simulink model "Model"  (R2019b)
settings: Solver=VariableStepAuto  StartTime=0.0  StopTime=10  RelTol=1e-3
values from neighbouring files (symbols this model uses):
  A = [u_j ; v_j ; w_j ; p_j ; q_j ; r_j ; x_j ; y_j ; z_j ; phi_j ; theta_j ; psi_j]    [LimSim7.m]
  B = [u_j ; v_j ; w_j ; p_j ; q_j ; r_j ; x_j ; y_j ; z_j ; phi_j ; theta_j ; psi_j]    [LimSim7.m]
  C = [h_j ; ax_j ; ay_j ; az_j]    [LimSim7.m]
  D = [h_j ; ax_j ; ay_j ; az_j]    [LimSim7.m]
  K_R = lqr(A_R, B_R, Q_R, R_R)    [LimSim7.m]
  M = [1, 1,    1, -1 ... (first row only)    [LimSim7.m]
  R = diag([1])    [LimSim7.m]
  tau1 = 30/1000    (= 0.03)    [LimSim7.m]
  tau2 = 1/10    (= 0.1)    [LimSim7.m]
libraries: sharedutil x4, vrlib x2, aerolibutil x1, simulink x1
settings Model: Creator=ethan  LastModifiedBy=ethan

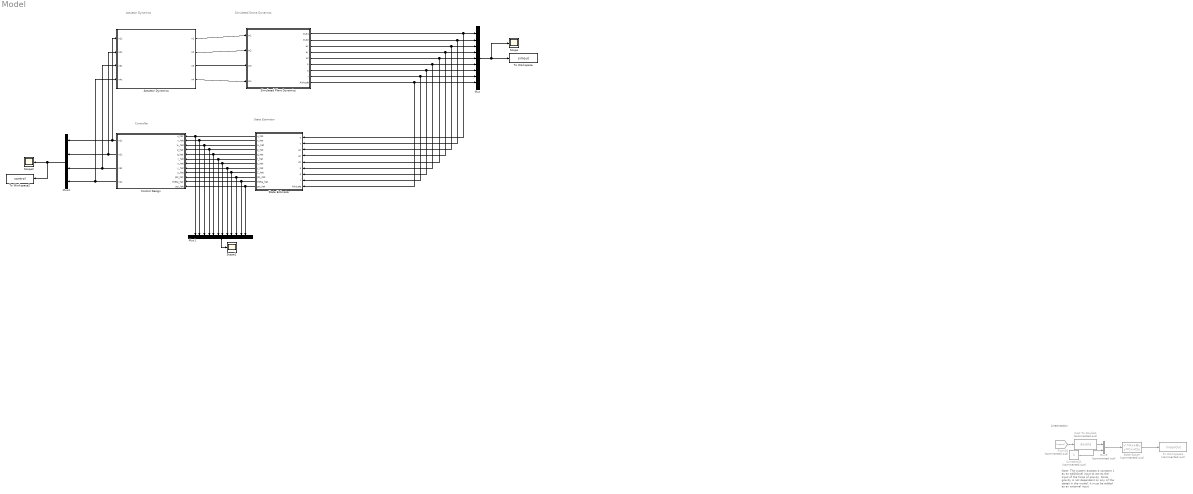
== system Model ==
  note: Actuator Dynamics
  note: Note: The system accepts a constant 1 as an additional input to act as the input of the force of gravity. Since gravity is not dependent on any of the states in the model, it must be added as an external input
  note: Linearization
  note: Simulated Drone Dynamics
  note: State Estimator
  note: Controller
  "Actuator Dynamics " : Subsystem
  Cast To Double1 : DataTypeConversion  Commented=on  OutDataTypeStr=double
  Constant21 : Constant  Commented=on
  Control Design : Subsystem
  From26 : From  Commented=on  GotoTag=motors
  Mux : Mux  Inputs=9
  Mux1 : Mux  Inputs=12
  Mux2 : Mux
  Mux9 : Mux  Commented=on  Inputs=2
  Scope : Scope
  Scope1 : Scope
  Scope2 : Scope
  Simulated Plant Dynamics : Subsystem
  State Estimator : Subsystem
  State-Space : StateSpace  Commented=on  A=A  B=B  C=C  D=D  InitialCondition=[0,0,0,0,0,0,0,0,0,0,0,0]
  To Workspace : ToWorkspace  VariableName=simout  SaveFormat=Structure With Time  SampleTime=-1
  To Workspace1 : ToWorkspace  Commented=on  VariableName=linearOut  SaveFormat=Timeseries  SampleTime=-1
  To Workspace2 : ToWorkspace  VariableName=control  SaveFormat=Timeseries  SampleTime=-1
  wires:
  State-Space/1 -> To Workspace1/1
  Constant21/1 -> Mux9/2
  Cast To Double1/1 -> Mux9/1
  From26/1 -> Cast To Double1/1
  Mux9/1 -> State-Space/1
  "Actuator Dynamics "/2(n2) -> Simulated Plant Dynamics/2(In2)
  "Actuator Dynamics "/1(n1) -> Simulated Plant Dynamics/1(In1)
  "Actuator Dynamics "/3(n3) -> Simulated Plant Dynamics/3(In3)
  "Actuator Dynamics "/4(n4) -> Simulated Plant Dynamics/4(In4)
  Simulated Plant Dynamics/1(Out1) -> Mux/1, State Estimator/1(u)
  Simulated Plant Dynamics/2(Out2) -> Mux/2, State Estimator/2(v)
  Simulated Plant Dynamics/3(ax) -> Mux/3, State Estimator/3(ax)
  Simulated Plant Dynamics/4(ay) -> Mux/4, State Estimator/4(ay)
  Simulated Plant Dynamics/5(az) -> State Estimator/5(az), Mux/5
  Simulated Plant Dynamics/6(p) -> State Estimator/6(p), Mux/6
  Simulated Plant Dynamics/7(q) -> Mux/7, State Estimator/7(q)
  Simulated Plant Dynamics/8(r) -> State Estimator/8(r), Mux/8
  Simulated Plant Dynamics/9(Altitude) -> State Estimator/9(Altitude), Mux/9
  State Estimator/1(u_hat) -> Mux1/1, Control Design/1(u_hat)
  State Estimator/2(v_hat) -> Mux1/2, Control Design/2(v_hat)
  State Estimator/3(w_hat) -> Control Design/3(w_hat), Mux1/3
  State Estimator/4(p_hat) -> Control Design/4(p_hat), Mux1/4
  State Estimator/5(q_hat) -> Control Design/5(q_hat), Mux1/5
  State Estimator/6(r_hat) -> Mux1/6, Control Design/6(r_hat)
  State Estimator/7(x_hat) -> Mux1/7, Control Design/7(x_hat)
  State Estimator/8(y_hat) -> Mux1/8, Control Design/8(y_hat)
  State Estimator/9(Z_hat) -> Mux1/9, Control Design/9(z_hat)
  State Estimator/10(phi_hat) -> Mux1/10, Control Design/10(phi_hat)
  State Estimator/11(theta_hat) -> Control Design/11(theta_hat), Mux1/11
  State Estimator/12(psi_hat) -> Control Design/12(psi_hat), Mux1/12
  Control Design/1(n1c) -> "Actuator Dynamics "/1(n1c), Mux2/1
  Control Design/2(n2c) -> "Actuator Dynamics "/2(n2c), Mux2/2
  Control Design/3(n3c) -> "Actuator Dynamics "/3(n3c), Mux2/3
  Control Design/4(n4c) -> Mux2/4, "Actuator Dynamics "/4(n4c)
  Mux/1 -> Scope/1, To Workspace/1
  Mux1/1 -> Scope1/1
  Mux2/1 -> To Workspace2/1, Scope2/1

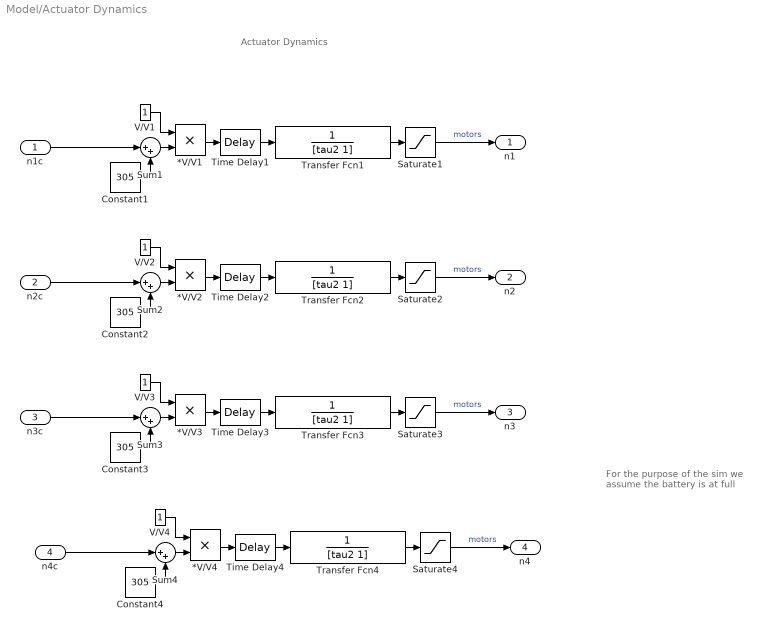
== system Model/Actuator Dynamics  ==
  note: For the purpose of the sim we assume the battery is at full
  note: Actuator Dynamics
  n1c : Inport
  n2c : Inport  Port=2
  n3c : Inport  Port=3
  n4c : Inport  Port=4
  *V/V{1..4} (4 alike) : Product
  Constant{1..4} (4 alike) : Constant  Value=305
  Saturate{1..4} (4 alike) : Saturate  UpperLimit=500  LowerLimit=10  OutDataTypeStr=single
  Sum{1..4} (4 alike) : Sum  Inputs=|++
  Time Delay{1..4} (4 alike) : TransportDelay  DelayTime=tau1
  Transfer Fcn{1..4} (4 alike) : TransferFcn  Denominator=[tau2 1]
  V/V{1..4} (4 alike) : Constant
  n1 : Outport
  n2 : Outport  Port=2
  n3 : Outport  Port=3
  n4 : Outport  Port=4
  wires:
  Transfer Fcn1/1 -> Saturate1/1
  n1c/1 -> Sum1/1
  Time Delay1/1 -> Transfer Fcn1/1
  Constant1/1 -> Sum1/2
  *V/V1/1 -> Time Delay1/1
  Sum1/1 -> *V/V1/2
  Saturate1/1 -> n1/1  "motors"
  V/V1/1 -> *V/V1/1
  Time Delay2/1 -> Transfer Fcn2/1
  Transfer Fcn2/1 -> Saturate2/1
  Constant2/1 -> Sum2/2
  Saturate2/1 -> n2/1  "motors"
  V/V2/1 -> *V/V2/1
  Sum2/1 -> *V/V2/2
  *V/V2/1 -> Time Delay2/1
  n2c/1 -> Sum2/1
  Time Delay3/1 -> Transfer Fcn3/1
  Transfer Fcn3/1 -> Saturate3/1
  Constant3/1 -> Sum3/2
  Saturate3/1 -> n3/1  "motors"
  V/V3/1 -> *V/V3/1
  Sum3/1 -> *V/V3/2
  *V/V3/1 -> Time Delay3/1
  n3c/1 -> Sum3/1
  Time Delay4/1 -> Transfer Fcn4/1
  Transfer Fcn4/1 -> Saturate4/1
  Constant4/1 -> Sum4/2
  Saturate4/1 -> n4/1  "motors"
  V/V4/1 -> *V/V4/1
  Sum4/1 -> *V/V4/2
  *V/V4/1 -> Time Delay4/1
  n4c/1 -> Sum4/1

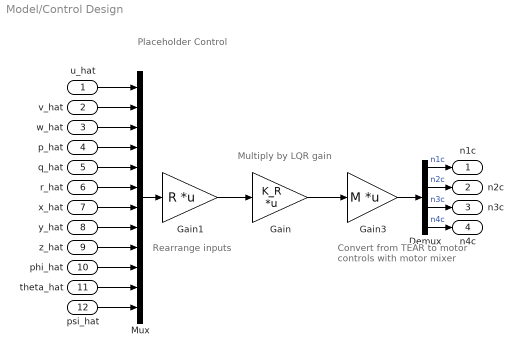
== system Model/Control Design ==
  note: Rearrange inputs
  note: Placeholder Control
  note: Multiply by LQR gain
  note: Convert from TEAR to motor controls with motor mixer
  u_hat : Inport
  v_hat : Inport  Port=2
  w_hat : Inport  Port=3
  p_hat : Inport  Port=4
  q_hat : Inport  Port=5
  r_hat : Inport  Port=6
  x_hat : Inport  Port=7
  y_hat : Inport  Port=8
  z_hat : Inport  Port=9
  phi_hat : Inport  Port=10
  theta_hat : Inport  Port=11
  psi_hat : Inport  Port=12
  Demux : Demux
  Gain : Gain  Gain=K_R  Multiplication=Matrix(K*u)
  Gain1 : Gain  Gain=R  Multiplication=Matrix(K*u)
  Gain3 : Gain  Gain=M  Multiplication=Matrix(K*u)
  Mux : Mux  Inputs=12
  n1c : Outport
  n2c : Outport  Port=2
  n3c : Outport  Port=3
  n4c : Outport  Port=4
  wires:
  Demux/1 -> n1c/1  "n1c"
  Demux/4 -> n4c/1  "n4c"
  theta_hat/1 -> Mux/11
  x_hat/1 -> Mux/7
  y_hat/1 -> Mux/8
  q_hat/1 -> Mux/5
  w_hat/1 -> Mux/3
  Demux/2 -> n2c/1  "n2c"
  p_hat/1 -> Mux/4
  Demux/3 -> n3c/1  "n3c"
  r_hat/1 -> Mux/6
  z_hat/1 -> Mux/9
  u_hat/1 -> Mux/1
  v_hat/1 -> Mux/2
  phi_hat/1 -> Mux/10
  psi_hat/1 -> Mux/12
  Mux/1 -> Gain1/1
  Gain1/1 -> Gain/1
  Gain/1 -> Gain3/1
  Gain3/1 -> Demux/1

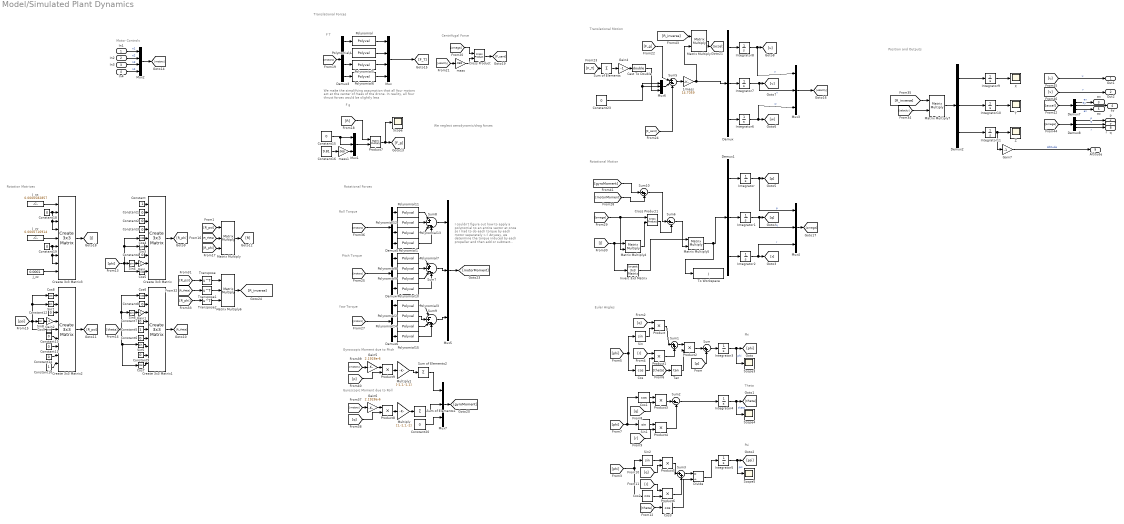
== system Model/Simulated Plant Dynamics ==
  note: I couldn't figure out how to apply a polynomial to an entire vector at once so I had to do each torque by each motor separately >:(
      |
      | Anyway, we determine the torque induced by each propeller and then add or subtract them accordingly to get the total torque about each axis
  note: We make the simplifying assumption that all four motors act at the center of mass of the drone. In reality, all four thrust forces would be slightly less
  note: Phi
  note: Motor Controls
  note: Translational Forces
  note: Euler Angles
  note: Rotation Matrices
  note: Theta
  note: Psi
  note: F g
  note: F T
  note: Translational Motion
  note: Rotational Motion
  note: Centrifugal Force
  note: Rotational Forces
  note: Pitch Torque
  note: Roll Torque
  note: Yaw Torque
  note: Gyroscopic Moment due to Pitch
  note: Gyroscopic Moment due to Roll
  note: Position and Outputs
  note: We neglect aerodynamic/drag forces
  In1 : Inport
  In2 : Inport  Port=2
  In3 : Inport  Port=3
  In4 : Inport  Port=4
  1/mass : Gain  Gain=14.7059
  Cast To Double : DataTypeConversion  OutDataTypeStr=double
  Constant : Constant
  Constant{1..4,6..9,11..15,18..20,23} (17 alike) : Constant  Value=0
  Constant10 : Constant
  Constant16 : Constant  Value=9.81
  Constant5 : Constant
  Cos{,1..9} (10 alike) : Trigonometry  Operator=cos
  Create 3x3 Matrix{,1..3} (4 alike) : sharedutil/Create 3x3 Matrix  aMode=aMode
  Cross Product : vrlib/Utilities/Cross Product
      settings: SourceProductName=Simulink
  Cross Product1 : vrlib/Utilities/Cross Product
      settings: SourceProductName=Simulink
  Demux{,1..2,7..8} (5 alike) : Demux  Outputs=3
  Demux{3..6} (4 alike) : Demux
  Divide : Product  Inputs=*/
  Gain{,1..2,4,7} (5 alike) : Gain  Gain=-1
  Gain5 : Gain  Gain=2.1928e-6
  Gain6 : Gain  Gain=2.1928e-6
  Integrator : Integrator  InitialCondition=rand/100
  Integrator{1..11} (11 alike) : Integrator
  Invert 3x3 Matrix : aerolibutil/Invert  3x3 Matrix
  J_xx : Constant  Value=0.0000582857
  J_yy : Constant  Value=0.0000716914
  J_zz : Constant  Value=0.0001
  Matrix Multiply : Product  Inputs=3  Multiplication=Matrix(*)
  Matrix Multiply{1,4..5,7} (4 alike) : Product  Multiplication=Matrix(*)
  Matrix Multiply6 : Product  Inputs=3  Multiplication=Matrix(*)
  Multiply : Gain  Gain=[1,-1,1,-1]
  Multiply1 : Gain  Gain=[-1,1,-1,1]
  Mux : Mux
  Mux{1,3..7} (6 alike) : Mux  Inputs=3
  Mux2 : Mux
  Polynomial{,4..6} (4 alike) : Polyval  Coefs=[ 1.066e-9 1.468e-6 0 0]
  Polynomial{1,7..13} (8 alike) : Polyval  Coefs=[ 5.07683e-11 6.99135e-8 0 0 ]
  Polynomial{2..3,14..15} (4 alike) : Polyval  Coefs="[  8.890e-9 0 0 ]"
  Product{,1..6,8..9} (9 alike) : Product
  Product7 : Product  Multiplication=Matrix(*)
  Scope{,3..5} (4 alike) : Scope
  Sin{,1..8} (9 alike) : Trigonometry
  Sum{,1,3,10} (4 alike) : Sum  Inputs=|++
  Sum of Elements : Sum  Inputs=+
  Sum of Elements1 : Sum  Inputs=+
  Sum of Elements2 : Sum  Inputs=+
  Sum2 : Sum  Inputs=|+-
  Sum5 : Sum  Inputs=|++-
  Sum6 : Sum  Inputs=|+-
  Sum7 : Sum  Inputs=|++--
  Sum8 : Sum  Inputs=|+--+
  Sum9 : Sum  Inputs=|-+-+
  Tan : Trigonometry  Operator=tan
  To Workspace : ToWorkspace  VariableName=j  SaveFormat=Structure  SampleTime=-1
  Transpose : Math  Operator=transpose  SignedPower=off  SaturateOnIntegerOverflow=on
  Transpose1 : Math  Operator=transpose  SignedPower=off  SaturateOnIntegerOverflow=on
  Transpose2 : Math  Operator=transpose  SignedPower=off  SaturateOnIntegerOverflow=on
  X : Scope
  Y : Scope
  Z : Scope
  mass : Gain  Gain=.068
  mass1 : Gain  Gain=.068
  Out1 : Outport
  Out2 : Outport  Port=2
  ax : Outport  Port=3
  ay : Outport  Port=4
  az : Outport  Port=5
  p : Outport  Port=6
  q : Outport  Port=7
  r : Outport  Port=8
  Altitude : Outport  Port=9
  wires:
  [omega] -> Demux8/1
  Product1/1 -> Sum1/2
  Polynomial7/1 -> Sum7/1
  Demux8/2 -> q/1  "q"
  Demux7/1 -> ax/1  "ax"
  In1/1 -> Mux2/1  "n1"
  Sin7/1 -> Create 3x3 Matrix2/2
  Integrator5/1 -> Scope5/1, [psi]  "psi"
  Sum10/1 -> Sum6/1
  [phi] -> Cos5/1, Cos4/1, Sin3/1, Sin4/1
  Gain4/1 -> Cast To Double/1
  Sum8/1 -> Mux5/1
  Create 3x3 Matrix/1 -> [R_phi]
  Integrator8/1 -> Mux3/1, [u]  "u"
  Constant5/1 -> Create 3x3 Matrix1/5
  Polynomial/1 -> Mux/1
  [phi] -> Cos/1, Sin/1
  Sum7/1 -> Mux5/2
  Constant20/1 -> Mux7/3
  Sin5/1 -> Create 3x3 Matrix1/7
  Demux5/3 -> Polynomial13/1
  Demux3/2 -> Polynomial4/1
  Product6/1 -> Sum3/2
  In4/1 -> Mux2/4  "n4"
  [phi] -> Sin1/1, Cos1/1
  Matrix Multiply1/1 -> [accel]
  Demux7/2 -> ay/1  "ay"
  Cos2/1 -> Product6/2
  Constant4/1 -> Create 3x3 Matrix/7
  Mux1/1 -> Product7/2
  Sin8/1 -> Gain2/1
  [v] -> Out2/1  "v"
  [F_cent] -> Sum5/3
  [theta] -> Cos6/1, Sin6/1, Cos7/1, Sin5/1
  Create 3x3 Matrix2/1 -> [R_psi]
  Product4/1 -> Sum2/2
  Polynomial13/1 -> Sum8/3
  Polynomial15/1 -> Sum9/4
  Constant3/1 -> Create 3x3 Matrix/4
  [p] -> Sum/2
  Product8/1 -> Multiply/1
  Constant13/1 -> Create 3x3 Matrix2/6
  Constant15/1 -> Mux1/2, Mux1/1
  Integrator6/1 -> Mux3/3, [w]  "w"
  Constant/1 -> Create 3x3 Matrix/1
  [r] -> Product4/2
  Constant9/1 -> Create 3x3 Matrix1/8
  1/mass/1 -> Matrix Multiply1/2, Demux/1
  [psi] -> Cos9/1, Cos8/1, Sin7/1, Sin8/1
  Constant2/1 -> Create 3x3 Matrix/3
  Product3/1 -> Sum2/1
  Integrator4/1 -> Scope4/1, [theta]  "theta"
  Sum5/1 -> 1/mass/1
  Cos6/1 -> Create 3x3 Matrix1/1
  Cos1/1 -> Product3/1
  [q] -> Product3/2
  [phi] -> Sin2/1, Cos2/1
  [q] -> Product8/2
  Integrator/1 -> Mux4/1, [p]  "p"
  Sin3/1 -> Create 3x3 Matrix/6
  Sum1/1 -> Product2/1
  [r] -> Product6/1
  Demux7/3 -> az/1  "az"
  Constant16/1 -> mass1/1
  [motors] -> Gain5/1
  Demux4/4 -> Polynomial10/1
  [q] -> Product5/2
  [motors] -> Demux6/1
  Sum of Elements/1 -> Gain4/1
  [theta] -> Cos3/1
  Integrator1/1 -> Mux4/2, [q]  "q"
  Sin6/1 -> Gain1/1
  Sum3/1 -> Divide/1
  Cos8/1 -> Create 3x3 Matrix2/1
  Constant1/1 -> Create 3x3 Matrix/2
  Product2/1 -> Sum/1
  Gain/1 -> Create 3x3 Matrix/8
  Integrator2/1 -> Mux4/3, [r]  "r"
  Transpose2/1 -> Matrix Multiply6/3
  J_yy/1 -> Create 3x3 Matrix3/5
  Product5/1 -> Sum3/1
  Integrator3/1 -> Scope3/1, [phi]  "phi"
  Gain1/1 -> Create 3x3 Matrix1/3
  Constant8/1 -> Create 3x3 Matrix1/2
  Gain6/1 -> Product8/1
  [R] -> Product7/1
  [R_phi] -> Matrix Multiply/3
  Constant14/1 -> Create 3x3 Matrix2/8
  Polynomial3/1 -> Sum9/1
  Matrix Multiply5/1 -> To Workspace/1, Demux1/1
  [R_psi] -> Matrix Multiply/1
  Cross Product/1 -> [F_cent]
  Matrix Multiply/1 -> [R]
  Constant10/1 -> Create 3x3 Matrix2/9
  Sin4/1 -> Gain/1
  Demux/3 -> Integrator6/1
  [theta] -> Tan/1
  Cos9/1 -> Create 3x3 Matrix2/5
  Sum2/1 -> Integrator4/1
  Mux4/1 -> [omega]
  Matrix Multiply7/1 -> Demux2/1
  Product/1 -> Sum1/1
  Gain2/1 -> Create 3x3 Matrix2/4
  Mux3/1 -> [velocity]
  Constant19/1 -> Create 3x3 Matrix3/8, Create 3x3 Matrix3/7, Create 3x3 Matrix3/6
  Polynomial6/1 -> Mux/4
  Polynomial1/1 -> Sum8/4
  [omega] -> Cross Product/1
  J_xx/1 -> Create 3x3 Matrix3/1
  J_zz/1 -> Create 3x3 Matrix3/9
  Sin2/1 -> Product5/1
  Product7/1 -> Scope/1, [F_g]
  Create 3x3 Matrix3/1 -> [J]
  [q] -> Product/1
  [R_theta] -> Transpose1/1
  Cos7/1 -> Create 3x3 Matrix1/9
  Multiply/1 -> Sum of Elements1/1
  Matrix Multiply6/1 -> [R_inverse]
  [F_g] -> Sum5/1
  Polynomial9/1 -> Sum7/3
  [R_phi] -> Transpose2/1
  Cos4/1 -> Create 3x3 Matrix/5
  Demux1/2 -> Integrator1/1
  [motorMoment] -> Sum10/2
  [r] -> Product1/1
  Invert 3x3 Matrix/1 -> Matrix Multiply5/1
  Constant12/1 -> Create 3x3 Matrix2/3
  Demux2/3 -> Integrator11/1
  Constant6/1 -> Create 3x3 Matrix1/6
  Demux3/3 -> Polynomial5/1
  [R_inverse] -> Matrix Multiply7/1
  Polynomial4/1 -> Mux/2
  [accel] -> Demux7/1
  Constant7/1 -> Create 3x3 Matrix1/4
  [velocity] -> mass/1
  Demux/1 -> Integrator8/1
  Mux/1 -> [F_T]
  Demux8/1 -> p/1  "p"
  [motors] -> Demux3/1
  Matrix Multiply4/1 -> Cross Product1/2
  Demux4/3 -> Polynomial9/1
  Create 3x3 Matrix1/1 -> [R_theta]
  Demux3/1 -> Polynomial/1
  Integrator10/1 -> Y/1
  Demux3/4 -> Polynomial6/1
  Transpose1/1 -> Matrix Multiply6/2
  Cast To Double/1 -> Mux6/3
  [velocity] -> Matrix Multiply7/2
  [F_T] -> Sum of Elements/1
  Demux1/3 -> Integrator2/1
  Mux6/1 -> Sum5/2
  [R_inverse] -> Matrix Multiply1/1
  [motors] -> Demux4/1
  Polynomial10/1 -> Sum7/4
  Sum/1 -> Integrator3/1
  In2/1 -> Mux2/2  "n2"
  Sin/1 -> Product/2
  Polynomial14/1 -> Sum9/3
  Integrator7/1 -> Mux3/2, [v]  "v"
  Demux5/4 -> Polynomial1/1
  Sin1/1 -> Product4/1
  Demux8/3 -> r/1  "r"
  Demux5/1 -> Polynomial11/1
  Demux5/2 -> Polynomial12/1
  [motors] -> Demux5/1
  Demux6/4 -> Polynomial15/1
  mass1/1 -> Mux1/3
  Demux6/3 -> Polynomial14/1
  Cos/1 -> Product1/2
  Demux6/1 -> Polynomial3/1
  [J] -> Matrix Multiply4/1, Invert 3x3 Matrix/1
  Constant18/1 -> Create 3x3 Matrix3/4, Create 3x3 Matrix3/3, Create 3x3 Matrix3/2
  Polynomial5/1 -> Mux/3
  Sum9/1 -> Mux5/3
  Constant11/1 -> Create 3x3 Matrix2/7
  Product9/1 -> Multiply1/1
  [p] -> Product9/2
  Cos5/1 -> Create 3x3 Matrix/9
  Integrator11/1 -> Gain7/1, Z/1
  Demux6/2 -> Polynomial2/1
  Multiply1/1 -> Sum of Elements2/1
  [R_theta] -> Matrix Multiply/2
  [R_psi] -> Transpose/1
  Gain5/1 -> Product9/1
  Polynomial11/1 -> Sum8/1
  Demux4/2 -> Polynomial8/1
  Mux7/1 -> [gyroMoment]
  Cross Product1/1 -> Sum6/2
  Demux1/1 -> Integrator/1
  [omega] -> Matrix Multiply4/2, Cross Product1/1
  Sum of Elements2/1 -> Mux7/1
  mass/1 -> Cross Product/2
  Demux/2 -> Integrator7/1
  Sum of Elements1/1 -> Mux7/2
  [gyroMoment] -> Sum10/1
  Divide/1 -> Integrator5/1
  Demux2/1 -> Integrator9/1
  Transpose/1 -> Matrix Multiply6/1
  [motors] -> Gain6/1
  Cos3/1 -> Divide/2
  Tan/1 -> Product2/2
  Mux5/1 -> [motorMoment]
  Demux2/2 -> Integrator10/1
  Polynomial12/1 -> Sum8/2
  Constant23/1 -> Mux6/1, Mux6/2
  Integrator9/1 -> X/1
  Polynomial2/1 -> Sum9/2
  Demux4/1 -> Polynomial7/1
  Sum6/1 -> Matrix Multiply5/2
  Polynomial8/1 -> Sum7/2
  In3/1 -> Mux2/3  "n3"
  Gain7/1 -> Altitude/1  "Altitude"
  [u] -> Out1/1  "u"
  Mux2/1 -> [motors]

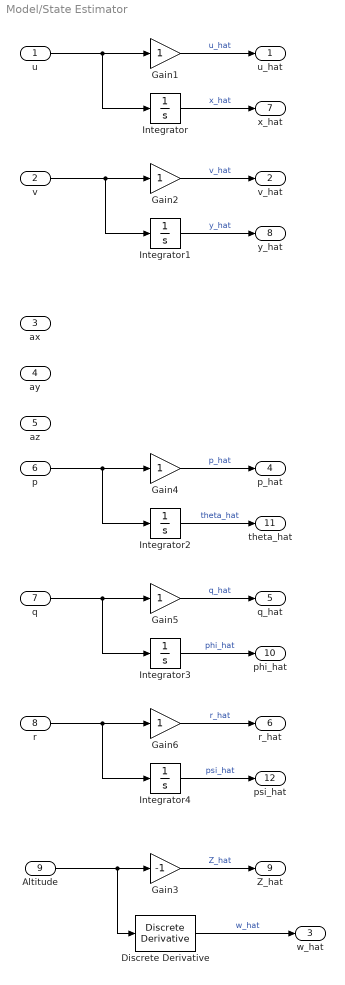
== system Model/State Estimator ==
  u : Inport
  v : Inport  Port=2
  ax : Inport  Port=3
  ay : Inport  Port=4
  az : Inport  Port=5
  p : Inport  Port=6
  q : Inport  Port=7
  r : Inport  Port=8
  Altitude : Inport  Port=9
  Discrete Derivative : simulink/Discrete/Discrete Derivative  gainval=1.0  ICPrevScaledInput=0.0  OutMin=[]  OutMax=[]  OutDataType=fixdt(1, 16)  OutScaling=2^-10  DoSatur=off
  Gain{1..2,4..6} (5 alike) : Gain
  Gain3 : Gain  Gain=-1
  Integrator{,1..4} (5 alike) : Integrator
  u_hat : Outport
  v_hat : Outport  Port=2
  w_hat : Outport  Port=3
  p_hat : Outport  Port=4
  q_hat : Outport  Port=5
  r_hat : Outport  Port=6
  x_hat : Outport  Port=7
  y_hat : Outport  Port=8
  Z_hat : Outport  Port=9
  phi_hat : Outport  Port=10
  theta_hat : Outport  Port=11
  psi_hat : Outport  Port=12
  wires:
  Gain5/1 -> q_hat/1  "q_hat"
  r/1 -> Integrator4/1, Gain6/1
  Integrator3/1 -> phi_hat/1  "phi_hat"
  Gain6/1 -> r_hat/1  "r_hat"
  q/1 -> Integrator3/1, Gain5/1
  u/1 -> Integrator/1, Gain1/1
  Gain3/1 -> Z_hat/1  "Z_hat"
  v/1 -> Integrator1/1, Gain2/1
  Altitude/1 -> Discrete Derivative/1, Gain3/1
  p/1 -> Integrator2/1, Gain4/1
  Integrator/1 -> x_hat/1  "x_hat"
  Integrator4/1 -> psi_hat/1  "psi_hat"
  Integrator1/1 -> y_hat/1  "y_hat"
  Discrete Derivative/1 -> w_hat/1  "w_hat"
  Gain2/1 -> v_hat/1  "v_hat"
  Gain1/1 -> u_hat/1  "u_hat"
  Gain4/1 -> p_hat/1  "p_hat"
  Integrator2/1 -> theta_hat/1  "theta_hat"
